simulink model "fullwave"  (R2021a)
settings: Solver=VariableStepAuto  StartTime=0.0  StopTime=10.0  RelTol=1e-3
libraries: spsDiodeLib x8, spsVoltageMeasurementLib x4, spsACVoltageSourceLib x2, spsGroundLib x2, spsLinearTransformerLib x2, spsSeriesRLCBranchLib x2, spspowerguiLib x2, spsParallelRLCBranchLib x1
settings Model: Creator=Aftab  LastModifiedBy=Aftab
settings DataIOCC: ReturnWorkspaceOutputs=off

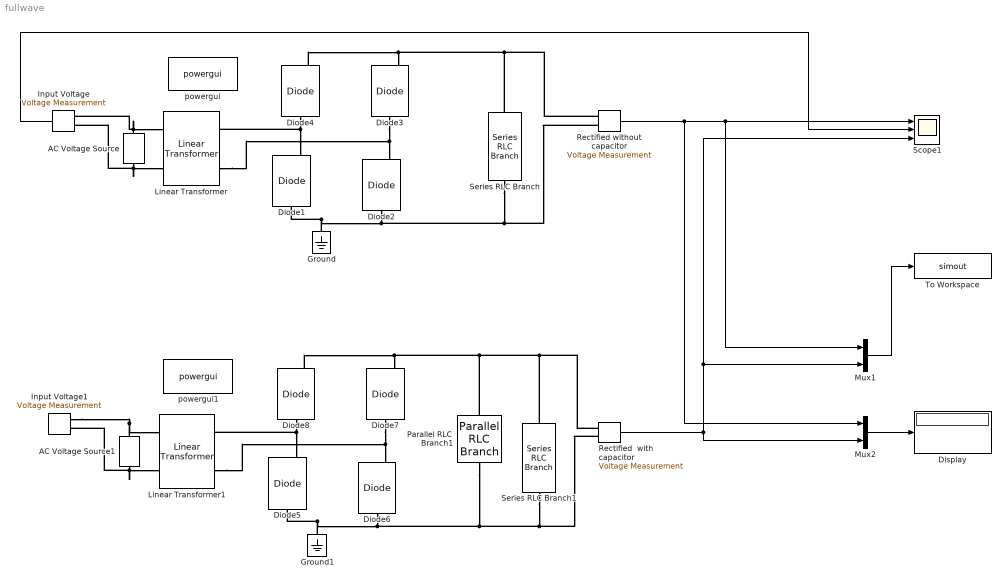
== system fullwave ==
  AC Voltage Source : spsACVoltageSourceLib/AC Voltage Source  Amplitude=220  Phase=0  Frequency=50  SampleTime=0  Measurements=None  BusType=swing  Pref=10e3  Qref=0  Qmin=-inf  Qmax=+inf
  AC Voltage Source1 : spsACVoltageSourceLib/AC Voltage Source  Amplitude=220  Phase=0  Frequency=50  SampleTime=0  Measurements=None  BusType=swing  Pref=10e3  Qref=0  Qmin=-inf  Qmax=+inf
  Diode{1..8} (8 alike) : spsDiodeLib/Diode  Ron=0.001  Lon=0  Vf=0.8  IC=0  UseSnubber=0  Rs=500  Cs=250e-9  Measurements=on
  Display : Display
  Ground : spsGroundLib/Ground  LConnTagsString=a
  Ground1 : spsGroundLib/Ground  LConnTagsString=a
  Input Voltage : spsVoltageMeasurementLib/Voltage Measurement  PhasorSimulation=off  OutputType=Complex  PSBequivalent=0
  Input Voltage1 : spsVoltageMeasurementLib/Voltage Measurement  PhasorSimulation=off  OutputType=Complex  PSBequivalent=0
  Linear Transformer : spsLinearTransformerLib/Linear Transformer  UNITS=SI  NominalPower=[ 250e6 50 ]  winding1=[220 0 0]  winding2=[9 0 0]  ThreeWindings=off  winding3=[3.15e+05 0.7938 0.084225]  RmLm=[500 500]  Measurements=None  DataType=on
  Linear Transformer1 : spsLinearTransformerLib/Linear Transformer  UNITS=SI  NominalPower=[ 250e6 50 ]  winding1=[220 0 0]  winding2=[9 0 0]  ThreeWindings=off  winding3=[3.15e+05 0.7938 0.084225]  RmLm=[500 500]  Measurements=None  DataType=on
  Mux1 : Mux  Inputs=2
  Mux2 : Mux  Inputs=2
  Parallel RLC Branch1 : spsParallelRLCBranchLib/Parallel RLC Branch  LConnTagsString=a  RConnTagsString=__new0  BranchType=C  Resistance=1  Inductance=1e-3  SetiL0=off  InitialCurrent=0  Capacitance=50  Setx0=off  InitialVoltage=0  Measurements=None
  Rectified  with capacitor : spsVoltageMeasurementLib/Voltage Measurement  PhasorSimulation=off  OutputType=Complex  PSBequivalent=0
  Rectified without capacitor : spsVoltageMeasurementLib/Voltage Measurement  PhasorSimulation=off  OutputType=Complex  PSBequivalent=0
  Scope1 : Scope  NumInputPorts=3
  Series RLC Branch : spsSeriesRLCBranchLib/Series RLC Branch  LConnTagsString=__new0  RConnTagsString=__new0  BranchType=R  Resistance=1  Inductance=1e-3  SetiL0=off  InitialCurrent=0  Capacitance=1e-6  Setx0=off  InitialVoltage=0  Measurements=None
  Series RLC Branch1 : spsSeriesRLCBranchLib/Series RLC Branch  LConnTagsString=__new0  RConnTagsString=__new0  BranchType=R  Resistance=1  Inductance=1e-3  SetiL0=off  InitialCurrent=0  Capacitance=1e-6  Setx0=off  InitialVoltage=0  Measurements=None
  To Workspace : ToWorkspace  VariableName=simout  SaveFormat=Timeseries  SampleTime=-1
      settings: Save2DSignal=2-D array (concatenate along first dimension)
  powergui : spspowerguiLib/powergui  Priority=1  SimulationMode=Continuous  SampleTime=50e-6  frequency=60  Iterations=50  frequencyindice=0  Pbase=100e6  ErrMax=1e-4  UnitsV=kV  UnitsW=MW  buscounter=0  FunctionMessages=off  echomessages=off  EnableUseOfTLC=off  CurrentSourceSwitches=off  DisableSnubberDevices=off  DisableRonSwitches=off  DisableVfSwitches=off  DisplayEquations=off  AutomaticDiscreteSolvers=off  SolverType=Tustin/Backward Euler (TBE)  Interpol=off  ExternalGateDelay=off  methode=off  Ts=100  x0status=blocks  SPID=on  SwTol=0  HookPort=off  NonlinearTolerance=1e-4  nMaxIteration=100  ContinueOnMaxIteration=off  RestoreLinks=warning  ResistiveCurrentMeasurement=off  Frange=[0:2:500]  Ylog=off  Xlog=on  ShowGrid=off  save=off  variable=ZData  structure=0  ZoomFFT=off  StartTime=0.0  cycles=1  DisplayStyle=1  fundamental=60  FreqAxis=off  MaxFrequency=1000  frequencyindicesteady=1  RmsSteady=1  display=off
  powergui1 : spspowerguiLib/powergui  Priority=1  SimulationMode=Continuous  SampleTime=50e-6  frequency=60  Iterations=50  frequencyindice=0  Pbase=100e6  ErrMax=1e-4  UnitsV=kV  UnitsW=MW  buscounter=0  FunctionMessages=off  echomessages=off  EnableUseOfTLC=off  CurrentSourceSwitches=off  DisableSnubberDevices=off  DisableRonSwitches=off  DisableVfSwitches=off  DisplayEquations=off  AutomaticDiscreteSolvers=off  SolverType=Tustin/Backward Euler (TBE)  Interpol=off  ExternalGateDelay=off  methode=off  Ts=100  x0status=blocks  SPID=on  SwTol=0  HookPort=off  NonlinearTolerance=1e-4  nMaxIteration=100  ContinueOnMaxIteration=off  RestoreLinks=warning  ResistiveCurrentMeasurement=off  Frange=[0:2:500]  Ylog=off  Xlog=on  ShowGrid=off  save=off  variable=ZData  structure=0  ZoomFFT=off  StartTime=0.0  cycles=1  DisplayStyle=1  fundamental=60  FreqAxis=off  MaxFrequency=1000  frequencyindicesteady=1  RmsSteady=1  display=off
  wires:
  Input Voltage/1 -> Scope1/2
  Rectified without capacitor/1 -> Mux2/1, Mux1/1, Scope1/1
  Rectified  with capacitor/1 -> Mux2/2, Scope1/3, Mux1/2
  Mux1/1 -> To Workspace/1
  Mux2/1 -> Display/1
  connections:
  AC Voltage Source/LConn1 -- Input Voltage/LConn1 -- Linear Transformer/LConn2
  Diode4/LConn1 -- Linear Transformer/RConn1 -- Diode1/RConn1
  Input Voltage/LConn2 -- AC Voltage Source/RConn1 -- Linear Transformer/LConn1
  Diode3/LConn1 -- Linear Transformer/RConn2 -- Diode2/RConn1
  Ground/LConn1 -- Rectified without capacitor/LConn2 -- Series RLC Branch/RConn1 -- Diode2/LConn1 -- Diode1/LConn1
  Rectified without capacitor/LConn1 -- Series RLC Branch/LConn1 -- Diode4/RConn1 -- Diode3/RConn1
  AC Voltage Source1/LConn1 -- Linear Transformer1/LConn2 -- Input Voltage1/LConn1
  Diode8/LConn1 -- Diode5/RConn1 -- Linear Transformer1/RConn1
  AC Voltage Source1/RConn1 -- Linear Transformer1/LConn1 -- Input Voltage1/LConn2
  Diode7/LConn1 -- Linear Transformer1/RConn2 -- Diode6/RConn1
  Ground1/LConn1 -- Diode5/LConn1 -- Series RLC Branch1/RConn1 -- Rectified  with capacitor/LConn2 -- Parallel RLC Branch1/LConn1 -- Diode6/LConn1
  Rectified  with capacitor/LConn1 -- Series RLC Branch1/LConn1 -- Parallel RLC Branch1/RConn1 -- Diode8/RConn1 -- Diode7/RConn1
